simulink model "hinf_arduino_condom"  (R2015a)
settings: Solver=ode3  StartTime=0.0  StopTime=10.0  FixedStep=1/200  RelTol=1e-3
values from neighbouring files (symbols this model uses):
  R = diag([0.00127,10e-9,10e-9])    [kalmanTest.m]
undefined symbols (not defined in the file or in its folder): Discrete, Hinf, Obs, Time
libraries: PoliArd x9, simulink x6, ctrlSharedLib x1
settings Model: ExtModeTrigDuration=2  Creator=GSavaia  LastModifiedBy=user
settings OptimizationCC: OptimizeModelRefInitCode=on  LifeSpan=1
settings DebuggingCC: UnderspecifiedInitializationDetection=Classic  MergeDetectMultiDrivingBlocksExec=none
settings HardwareCC: ProdLargestAtomicInteger=Long  ProdLargestAtomicFloat=Double  ProdEndianess=LittleEndian  ProdHWDeviceType=ARM Compatible->ARM Cortex
settings RTWCC: SystemTargetFile=realtime.tlc  GenerateMakefile=off  TemplateMakefile=realtime.tmf  Description=Run on Target Hardware  RTWVerbose=off
settings ERTTargetCC: CombineOutputUpdateFcns=off  ExtModeTransport=3  ExtModeMexFile=ext_serial_win32_comm_rtt  ExtModeMexArgs=0 1 9600  ERTSrcFileBannerTemplate=realtime_code_template.cgt  ERTHdrFileBannerTemplate=realtime_code_template.cgt  ERTDataSrcFileTemplate=realtime_code_template.cgt  ERTDataHdrFileTemplate=realtime_code_template.cgt  ERTCustomFileTemplate=realtime_file_process.tlc

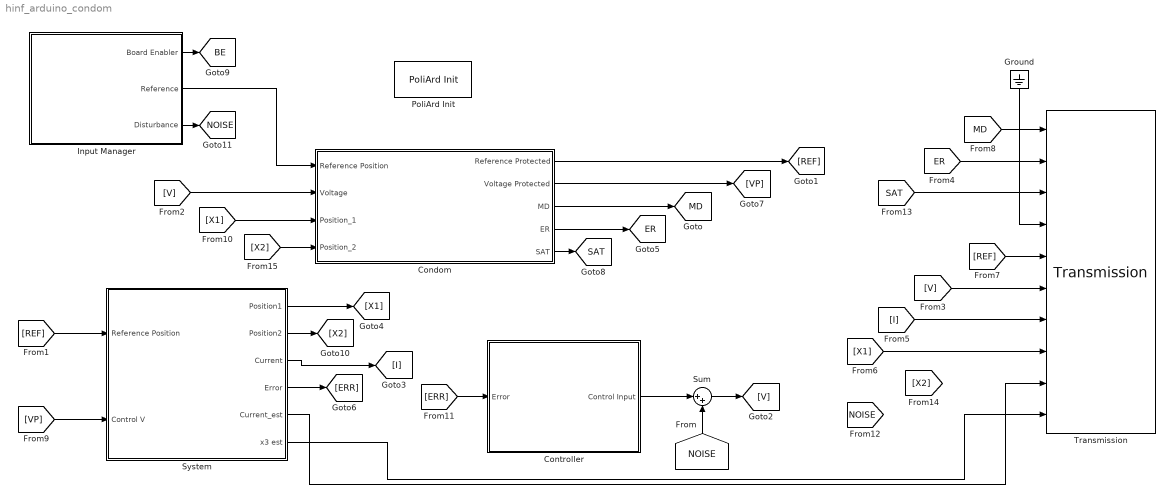
== system hinf_arduino_condom ==
  Condom : Subsystem
  Controller : Subsystem
  Ground : Ground
  Input Manager : Subsystem
  PoliArd Init : PoliArd/PoliArd Init
  Sum : Sum  Inputs=|++
  "System " : Subsystem
  Transmission : PoliArd/Transmission  sample_freq=200  sig_to_send=6
  tag scope: BE=global, ER=global, MD=global, NOISE=global, SAT=global
  wires:
  Condom/1(Reference Protected) -> [REF]
  [REF] -> "System "/1(Reference Position)
  "System "/3(Current) -> [I]
  [V] -> Condom/2(Voltage)
  [V] -> Transmission/6
  [I] -> Transmission/7
  "System "/1(Position1) -> [X1]
  [REF] -> Transmission/5
  [MD] -> Transmission/1
  [VP] -> "System "/2(Control V)
  [X1] -> Condom/3(Position_1)
  [X1] -> Transmission/8
  "System "/4(Error) -> [ERR]
  [ERR] -> Controller/1(Error)
  Condom/2("Voltage Protected ") -> [VP]
  Condom/3(MD) -> [MD]
  Condom/4(ER) -> [ER]
  Ground/1 -> Transmission/4
  [ER] -> Transmission/2
  [SAT] -> Transmission/3
  Condom/5(SAT) -> [SAT]
  Sum/1 -> [V]
  Controller/1(Control Input) -> Sum/1
  [NOISE] -> Sum/2
  Input Manager/1(Board Enabler) -> [BE]
  Input Manager/3(Disturbance) -> [NOISE]
  Input Manager/2(Reference) -> Condom/1(Reference Position)
  "System "/2(Position2) -> [X2]
  [X2] -> Condom/4(Position_2)
  "System "/6("x3 est ") -> Transmission/10
  "System "/5("Current_est ") -> Transmission/9

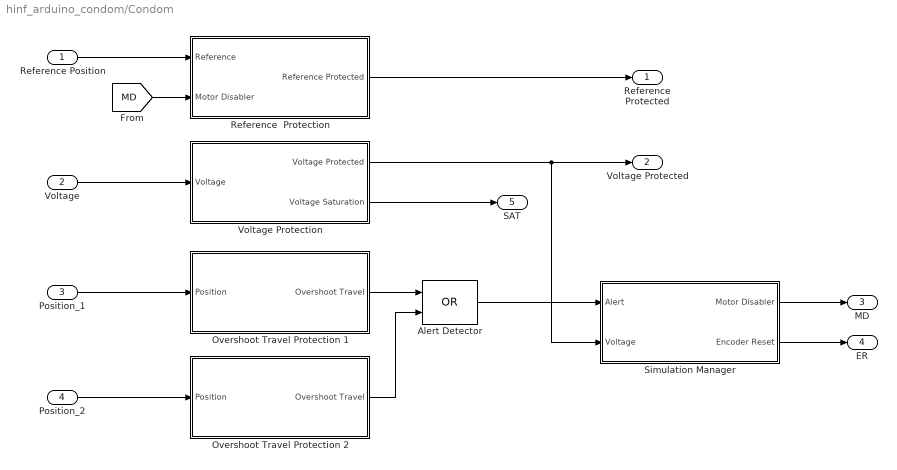
== system hinf_arduino_condom/Condom ==
  Reference Position : Inport
  Voltage : Inport  Port=2
  Position_1 : Inport  Port=3
  Position_2 : Inport  Port=4
  Alert Detector : Logic  Operator=OR  AllPortsSameDT=off  OutDataTypeStr=boolean
  Overshoot Travel Protection 1 : Subsystem
  Overshoot Travel Protection 2 : Subsystem
  Reference  Protection : Subsystem
  Simulation Manager : Subsystem
  Voltage Protection : Subsystem
  Reference Protected : Outport
  "Voltage Protected " : Outport  Port=2
  MD : Outport  Port=3
  ER : Outport  Port=4
  SAT : Outport  Port=5
  wires:
  Reference Position/1 -> Reference  Protection/1("Reference ")
  Position_1/1 -> Overshoot Travel Protection 1/1("Position ")
  Overshoot Travel Protection 1/1(Overshoot Travel) -> Alert Detector/1
  Voltage/1 -> Voltage Protection/1("Voltage ")
  Voltage Protection/1(Voltage Protected) -> Simulation Manager/2(Voltage), "Voltage Protected "/1
  Reference  Protection/1(Reference Protected) -> Reference Protected/1
  Alert Detector/1 -> Simulation Manager/1(Alert)
  Simulation Manager/2(Encoder Reset) -> ER/1
  Simulation Manager/1(Motor Disabler) -> MD/1
  [MD] -> Reference  Protection/2(Motor Disabler)
  Voltage Protection/2(Voltage Saturation) -> SAT/1
  Position_2/1 -> Overshoot Travel Protection 2/1("Position ")
  Overshoot Travel Protection 2/1(Overshoot Travel) -> Alert Detector/2

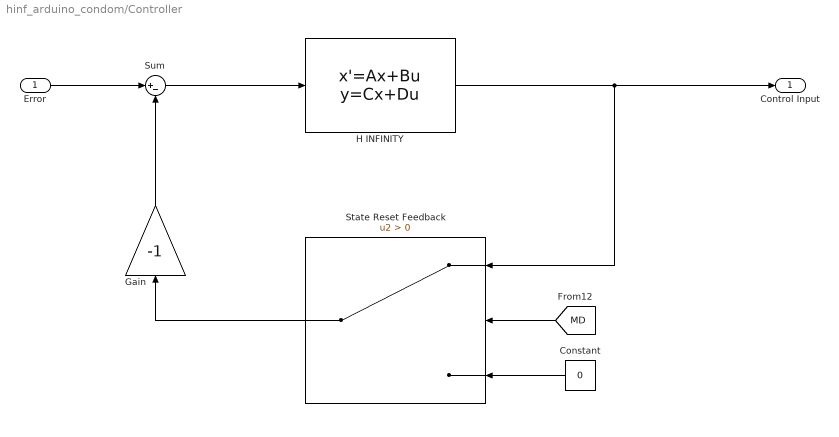
== system hinf_arduino_condom/Controller ==
  Error : Inport
  Constant : Constant  Value=0
  Gain : Gain  Gain=-1
  H INFINITY : StateSpace  A=Hinf.A  B=Hinf.B  C=Hinf.C  D=Hinf.D  X0=0
  State Reset Feedback : Switch  Criteria=u2 > Threshold
  Sum : Sum  Inputs=|+-
  Control Input : Outport
  wires:
  H INFINITY/1 -> State Reset Feedback/1, Control Input/1
  Error/1 -> Sum/1
  Sum/1 -> H INFINITY/1
  Constant/1 -> State Reset Feedback/3
  Gain/1 -> Sum/2
  State Reset Feedback/1 -> Gain/1
  [MD] -> State Reset Feedback/2

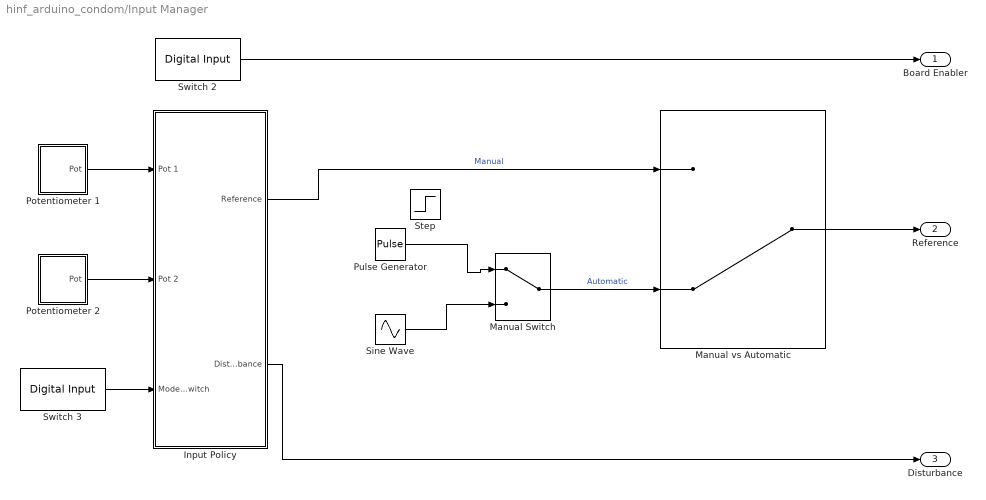
== system hinf_arduino_condom/Input Manager ==
  Input Policy : Subsystem
  Manual vs Automatic : ManualSwitch  CurrentSetting=0
  Manual Switch : ManualSwitch
  Potentiometer 1 : Subsystem
  Potentiometer 2 : Subsystem
  Pulse Generator : DiscretePulseGenerator  PulseType=Time based  Period=10  PulseWidth=50  PhaseDelay=5
  Sine Wave : Sin  Amplitude=0.5  Bias=0.7  Frequency=pi  SampleTime=0
  Step : Step  Time=5  SampleTime=0
  Switch 2 : PoliArd/Digital Input  DI_pin=2  DIsample=-1
  Switch 3 : PoliArd/Digital Input  DI_pin=3  DIsample=-1
  Board Enabler : Outport
  Reference : Outport  Port=2
  Disturbance : Outport  Port=3
  wires:
  Switch 2/1 -> Board Enabler/1
  Switch 3/1 -> Input Policy/3(Mode Switch)
  Sine Wave/1 -> Manual Switch/2
  Potentiometer 1/1(Pot) -> Input Policy/1(Pot 1)
  Potentiometer 2/1(Pot) -> Input Policy/2(Pot 2)
  Input Policy/1(Reference) -> Manual vs Automatic/1  "Manual"
  Manual Switch/1 -> Manual vs Automatic/2  "Automatic"
  Input Policy/2(Disturbance) -> Disturbance/1
  Manual vs Automatic/1 -> Reference/1
  Pulse Generator/1 -> Manual Switch/1

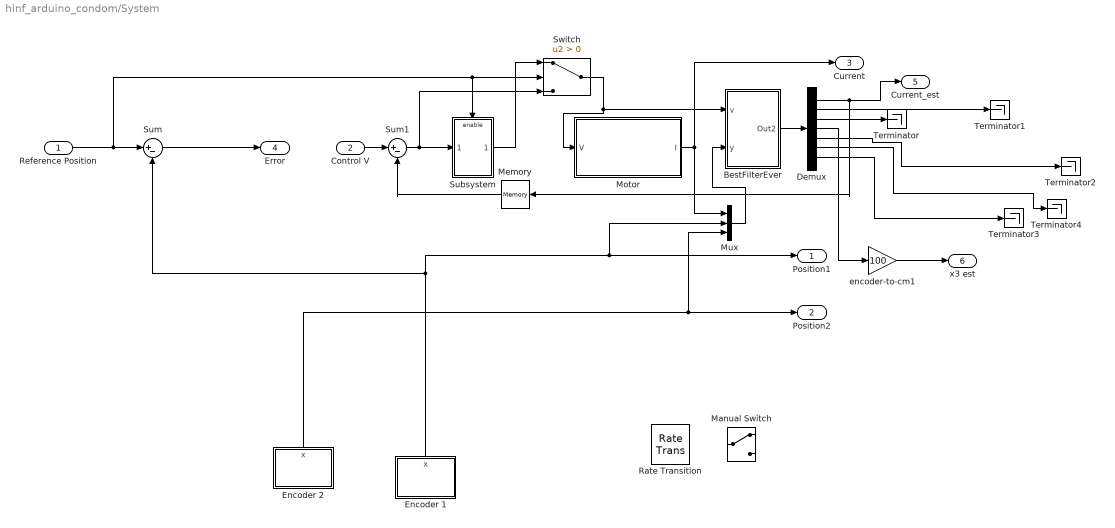
== system hinf_arduino_condom/System  ==
  Reference Position : Inport
  Control V : Inport  Port=2
  BestFilterEver : Subsystem
  Demux : Demux  Outputs=7
  "Encoder 1 " : Subsystem
  Encoder 2 : Subsystem
  Manual Switch : ManualSwitch
  Memory : Memory
  Motor : Subsystem
  Mux : Mux  Inputs=3
  Rate Transition : RateTransition
  Subsystem : Subsystem
  Sum : Sum  Inputs=|+-
  Sum1 : Sum  Inputs=|+-
  Switch : Switch  Criteria=u2 > Threshold
  Terminator{,1..4} (5 alike) : Terminator
  encoder-to-cm1 : Gain  Gain=100
  Position1 : Outport
  Position2 : Outport  Port=2
  Current : Outport  Port=3
  Error : Outport  Port=4
  "Current_est " : Outport  Port=5
  "x3 est " : Outport  Port=6
  wires:
  Reference Position/1 -> Switch/2, Subsystem/Enable, Sum/1
  Sum/1 -> Error/1
  Control V/1 -> Sum1/1
  Motor/1(I) -> Current/1, Mux/1
  BestFilterEver/1(Out2) -> Demux/1
  Mux/1 -> BestFilterEver/2(y)
  Demux/5 -> Terminator2/1
  Demux/6 -> Terminator4/1
  Demux/7 -> Terminator3/1
  "Encoder 1 "/1(x) -> Sum/2, Mux/2, Position1/1
  Demux/2 -> Terminator1/1
  Demux/4 -> encoder-to-cm1/1
  Demux/3 -> Terminator/1
  Demux/1 -> Memory/1, "Current_est "/1
  Switch/1 -> BestFilterEver/1(v), Motor/1(V)
  Subsystem/1(Out1) -> Switch/1
  encoder-to-cm1/1 -> "x3 est "/1
  Memory/1 -> Sum1/2
  Sum1/1 -> Switch/3, Subsystem/1(In1)
  Encoder 2/1(x) -> Mux/3, Position2/1

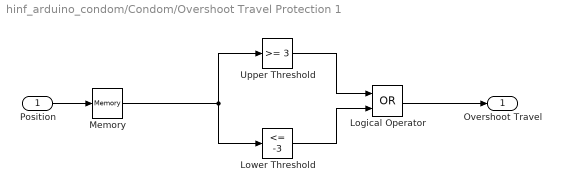
== system hinf_arduino_condom/Condom/Overshoot Travel Protection 1 ==
  "Position " : Inport
  Logical Operator : Logic  Operator=OR  AllPortsSameDT=off  OutDataTypeStr=boolean
  Lower Threshold : simulink/Logic and Bit Operations/Compare To Constant  relop=<=  const=-3  OutDataTypeStr=boolean
  Memory : Memory  InheritSampleTime=on
  Upper Threshold : simulink/Logic and Bit Operations/Compare To Constant  relop=>=  const=3  OutDataTypeStr=boolean
  Overshoot Travel : Outport
  wires:
  Logical Operator/1 -> Overshoot Travel/1
  Lower Threshold/1 -> Logical Operator/2
  Upper Threshold/1 -> Logical Operator/1
  "Position "/1 -> Memory/1
  Memory/1 -> Lower Threshold/1, Upper Threshold/1

== system hinf_arduino_condom/Condom/Overshoot Travel Protection 2 ==
  "Position " : Inport
  Logical Operator : Logic  Operator=OR  AllPortsSameDT=off  OutDataTypeStr=boolean
  Lower Threshold : simulink/Logic and Bit Operations/Compare To Constant  relop=<=  const=-3  OutDataTypeStr=boolean
  Memory : Memory  InheritSampleTime=on
  Upper Threshold : simulink/Logic and Bit Operations/Compare To Constant  relop=>=  const=3  OutDataTypeStr=boolean
  Overshoot Travel : Outport
  wires:
  Logical Operator/1 -> Overshoot Travel/1
  Lower Threshold/1 -> Logical Operator/2
  Upper Threshold/1 -> Logical Operator/1
  "Position "/1 -> Memory/1
  Memory/1 -> Lower Threshold/1, Upper Threshold/1

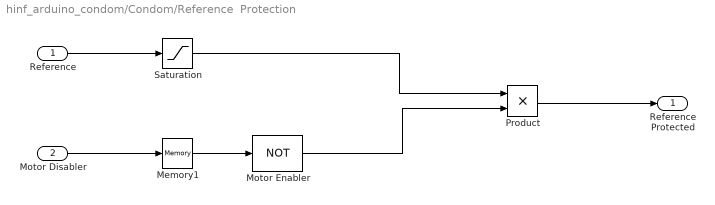
== system hinf_arduino_condom/Condom/Reference  Protection ==
  "Reference " : Inport
  Motor Disabler : Inport  Port=2
  Memory1 : Memory  X0=1  InheritSampleTime=on
  Motor Enabler : Logic  Operator=NOT  Inputs=1  AllPortsSameDT=off  OutDataTypeStr='double'
  Product : Product
  Saturation : Saturate  UpperLimit=3  LowerLimit=-3
  Reference Protected : Outport
  wires:
  "Reference "/1 -> Saturation/1
  Saturation/1 -> Product/1
  Motor Enabler/1 -> Product/2
  Memory1/1 -> Motor Enabler/1
  Product/1 -> Reference Protected/1
  Motor Disabler/1 -> Memory1/1

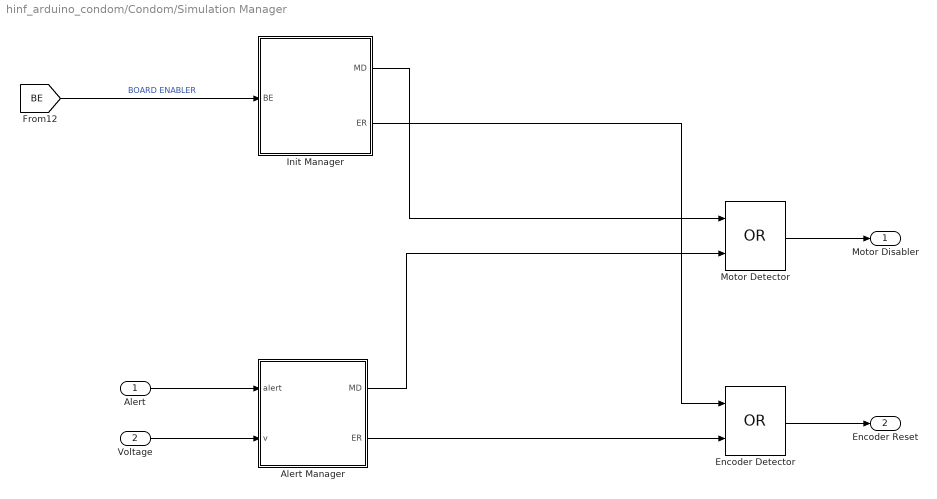
== system hinf_arduino_condom/Condom/Simulation Manager ==
  Alert : Inport
  Voltage : Inport  Port=2
  Alert Manager : Stateflow chart  TreatAsAtomicUnit=on
  Encoder Detector : Logic  Operator=OR  AllPortsSameDT=off  OutDataTypeStr=boolean
  Init Manager : Stateflow chart  TreatAsAtomicUnit=on
  Motor Detector : Logic  Operator=OR  AllPortsSameDT=off  OutDataTypeStr=boolean
  Motor Disabler : Outport
  Encoder Reset : Outport  Port=2
  wires:
  [BE] -> Init Manager/1(BE)  "BOARD ENABLER"
  Motor Detector/1 -> Motor Disabler/1
  Encoder Detector/1 -> Encoder Reset/1
  Init Manager/1(MD) -> Motor Detector/1
  Alert Manager/1(MD) -> Motor Detector/2
  Init Manager/2(ER) -> Encoder Detector/1
  Alert Manager/2(ER) -> Encoder Detector/2
  Alert/1 -> Alert Manager/1(alert)
  Voltage/1 -> Alert Manager/2(v)

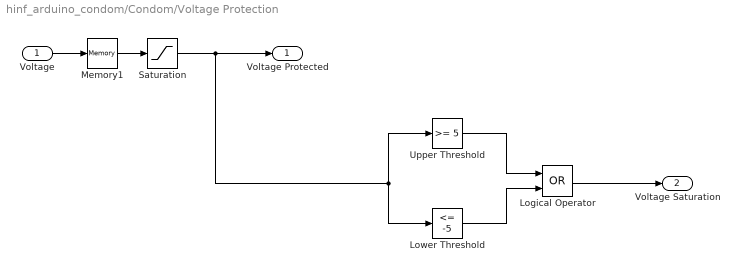
== system hinf_arduino_condom/Condom/Voltage Protection ==
  "Voltage " : Inport
  Logical Operator : Logic  Operator=OR  AllPortsSameDT=off  OutDataTypeStr=boolean
  Lower Threshold : simulink/Logic and Bit Operations/Compare To Constant  relop=<=  const=-5  OutDataTypeStr=boolean
  Memory1 : Memory  InheritSampleTime=on
  Saturation : Saturate  UpperLimit=5  LowerLimit=-5
  Upper Threshold : simulink/Logic and Bit Operations/Compare To Constant  relop=>=  const=5  OutDataTypeStr=boolean
  Voltage Protected : Outport
  Voltage Saturation : Outport  Port=2
  wires:
  "Voltage "/1 -> Memory1/1
  Logical Operator/1 -> Voltage Saturation/1
  Lower Threshold/1 -> Logical Operator/2
  Upper Threshold/1 -> Logical Operator/1
  Saturation/1 -> Lower Threshold/1, Upper Threshold/1, Voltage Protected/1
  Memory1/1 -> Saturation/1

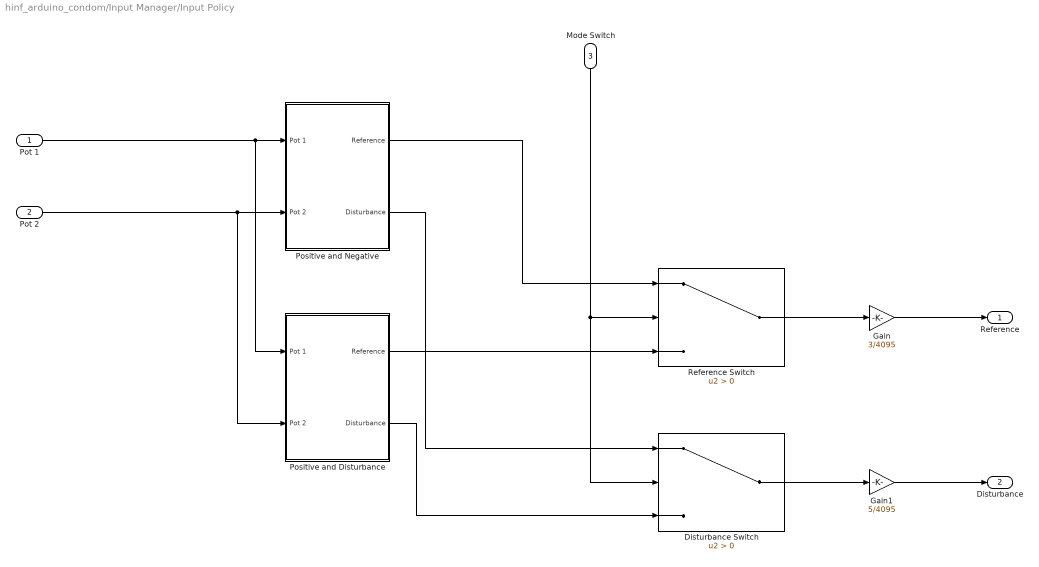
== system hinf_arduino_condom/Input Manager/Input Policy ==
  Pot 1 : Inport
  Pot 2 : Inport  Port=2
  Mode Switch : Inport  Port=3
  Disturbance Switch : Switch  Criteria=u2 > Threshold
  Gain : Gain  Gain=3/4095
  Gain1 : Gain  Gain=5/4095
  Positive and Disturbance : Subsystem
  Positive and Negative : Subsystem
  Reference Switch : Switch  Criteria=u2 > Threshold
  Reference : Outport
  Disturbance : Outport  Port=2
  wires:
  Pot 1/1 -> Positive and Disturbance/1(Pot 1), Positive and Negative/1(Pot 1)
  Pot 2/1 -> Positive and Disturbance/2(Pot 2), Positive and Negative/2(Pot 2)
  Mode Switch/1 -> Reference Switch/2, Disturbance Switch/2
  Reference Switch/1 -> Gain/1
  Disturbance Switch/1 -> Gain1/1
  Positive and Negative/1(Reference) -> Reference Switch/1
  Positive and Disturbance/1(Reference) -> Reference Switch/3
  Positive and Negative/2(Disturbance) -> Disturbance Switch/1
  Positive and Disturbance/2(Disturbance) -> Disturbance Switch/3
  Gain/1 -> Reference/1
  Gain1/1 -> Disturbance/1

== system hinf_arduino_condom/Input Manager/Potentiometer 1 ==
  Analog Input : PoliArd/Analog Input  AIpin_mask=8  AIsample=-1
  Data Type Conversion1 : DataTypeConversion
  Transfer Fcn : TransferFcn  Numerator=1  Denominator=[1/(2*pi*5) 1]
  Pot : Outport
  wires:
  Analog Input/1 -> Data Type Conversion1/1
  Transfer Fcn/1 -> Pot/1
  Data Type Conversion1/1 -> Transfer Fcn/1

== system hinf_arduino_condom/Input Manager/Potentiometer 2 ==
  Analog Input : PoliArd/Analog Input  AIpin_mask=9  AIsample=-1
  Data Type Conversion1 : DataTypeConversion
  Transfer Fcn : TransferFcn  Numerator=1  Denominator=[1/(2*pi*5) 1]
  Pot : Outport
  wires:
  Analog Input/1 -> Data Type Conversion1/1
  Transfer Fcn/1 -> Pot/1
  Data Type Conversion1/1 -> Transfer Fcn/1

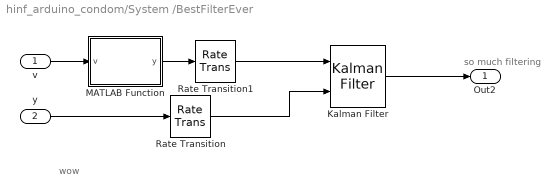
== system hinf_arduino_condom/System /BestFilterEver ==
  note: wow
  note: so much filtering
  v : Inport
  y : Inport  Port=2
  Kalman Filter : ctrlSharedLib/Kalman Filter  TimeDomain=Discrete-Time  UseCurrentEstimator=on  ModelSource=Individual A, B, C, D matrices  ModelSourceVariable=ss(0.95,1,1,0,1)  A=Obs.a  B=Obs.b  C=Obs.c  D=Obs.d  NumberOfStates=1  NumberOfInputs=1  NumberOfOutputs=1  InitialEstimateSource=Dialog  X0=0  P0=10  UseK=off  UseGH=off  NumberOfProcessNoiseInputs=1  G=1  TimeInvariantG=on  H=0  TimeInvariantH=on  Q=Q  TimeInvariantQ=on  R=R  TimeInvariantR=on  N=0  TimeInvariantN=on  AddInputPort=on  AddEnablePort=off  OutputEstimatedY=off  OutputP=off  Ts=1/200
  MATLAB Function : MATLAB Function  TreatAsAtomicUnit=on
  Rate Transition : RateTransition  OutPortSampleTime=1/200
  Rate Transition1 : RateTransition  OutPortSampleTime=1/200
  Out2 : Outport
  wires:
  y/1 -> Rate Transition/1
  Kalman Filter/1 -> Out2/1
  Rate Transition/1 -> Kalman Filter/2
  Rate Transition1/1 -> Kalman Filter/1
  v/1 -> MATLAB Function/1(v)
  MATLAB Function/1(y) -> Rate Transition1/1

== system hinf_arduino_condom/System /Encoder 1  ==
  Data Type Conversion1 : DataTypeConversion
  Encoder : PoliArd/Encoder  EncoderID=1  dt_enc=1/200
  encoder-to-cm : Gain  Gain=1/560
  x : Outport
  wires:
  Encoder/1 -> Data Type Conversion1/1
  [ER] -> Encoder/1
  encoder-to-cm/1 -> x/1
  Data Type Conversion1/1 -> encoder-to-cm/1

== system hinf_arduino_condom/System /Encoder 2 ==
  Data Type Conversion1 : DataTypeConversion
  Encoder : PoliArd/Encoder  EncoderID=4  dt_enc=1/200
  encoder-to-cm : Gain  Gain=1/560
  x : Outport
  wires:
  Encoder/1 -> Data Type Conversion1/1
  [ER] -> Encoder/1
  Data Type Conversion1/1 -> encoder-to-cm/1
  encoder-to-cm/1 -> x/1

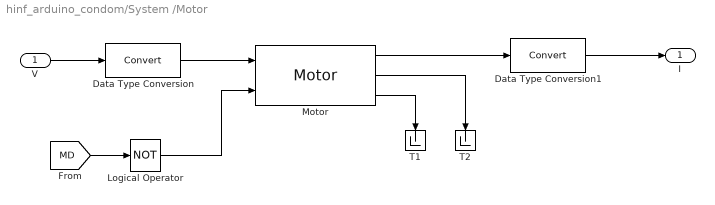
== system hinf_arduino_condom/System /Motor ==
  V : Inport
  Data Type Conversion : DataTypeConversion
  Data Type Conversion1 : DataTypeConversion
  Logical Operator : Logic  Operator=NOT  AllPortsSameDT=off  OutDataTypeStr=boolean
  Motor : PoliArd/Motor  MotorID=2  DC_bus_mask=12  dt_mot=1/200
  T1 : Terminator
  T2 : Terminator
  I : Outport
  wires:
  Data Type Conversion/1 -> Motor/1
  V/1 -> Data Type Conversion/1
  Motor/3 -> T1/1
  Motor/2 -> T2/1
  Motor/1 -> Data Type Conversion1/1
  Data Type Conversion1/1 -> I/1
  Logical Operator/1 -> Motor/2
  [MD] -> Logical Operator/1

== system hinf_arduino_condom/System /Subsystem ==
  In1 : Inport
  Enable : EnablePort
  Transfer Fcn : TransferFcn  Numerator=50  Denominator=[1 0]
  Out1 : Outport
  wires:
  Transfer Fcn/1 -> Out1/1
  In1/1 -> Transfer Fcn/1

== system hinf_arduino_condom/Input Manager/Input Policy/Positive and Disturbance ==
  Pot 1 : Inport
  Pot 2 : Inport  Port=2
  Reference : Outport
  Disturbance : Outport  Port=2
  wires:
  Pot 1/1 -> Reference/1
  Pot 2/1 -> Disturbance/1

== system hinf_arduino_condom/Input Manager/Input Policy/Positive and Negative ==
  Pot 1 : Inport
  Pot 2 : Inport  Port=2
  Add : Sum  Inputs=+-
  Constant : Constant  Value=0
  Reference : Outport
  Disturbance : Outport  Port=2
  wires:
  Add/1 -> Reference/1
  Constant/1 -> Disturbance/1
  Pot 2/1 -> Add/2
  Pot 1/1 -> Add/1

== stateflow chart hinf_arduino_condom/Condom/Simulation Manager/Init Manager ==
  state STOP
    entry:
    MD = 1;
    ER = 1;
  state OPERATIVE
    entry:
    MD = 0;
    ER = 0;
  state INIT
    entry:
    MD = 1;
    ER  = 1;
  (default) -> STOP
  OPERATIVE -> STOP : [BE==0]
  STOP -> INIT : [BE==1]
  INIT -> OPERATIVE : after(3, sec)
  data: MD output; ER output; BE input

== matlab function hinf_arduino_condom/System /BestFilterEver/MATLAB Function ==
  data: v input; y output
function y = fcn(v)

    if (v ==0)
        y=0;
    elseif (v>0)
        g=0.6564+0.1712*v-0.0317*v^2+0.0044*v^3;
        y = v.*g;
    else
        g=-0.21-1.1397*v-0.2756*v^2-0.0226*v^3;
        y = v.*g;
    end
end

== stateflow chart hinf_arduino_condom/Condom/Simulation Manager/Alert Manager ==
  state OK
    entry:
    MD=0;
    ER=0;
  state ALERT
    entry:
    MD=1;
    ER=1;
  (default) -> OK
  OK -> ALERT : [alert==1]
  ALERT -> OK : [abs(v)<0.3]
  data: alert input; v input; MD output; ER output
